simulink model "qpsk_phase_uw"  (R2016b)
settings: Solver=VariableStepAuto  StartTime=0.0  StopTime=(12+8+84)*8*4-1  RelTol=1e-3  EnableMultiTasking=on
undefined symbols (not defined in the file or in its folder): jsin, K1, K2, rcosine
libraries: dspstat3 x1
settings Model: Creator=coltmt  LastModifiedBy=colttom
settings DataIOCC: LimitDataPoints=on
settings OptimizationCC: LifeSpan=inf
settings DebuggingCC: AllowSymbolicDim=off  SFUnexpectedBacktrackingDiag=warning  SFNoUnconditionalDefaultTransitionDiag=warning  SFExecutionAtInitializationDiag=none
settings ModelReferenceCC: PropagateSignalLabelsOutOfModel=off
settings GRTTargetCC: TargetLangStandard=C89/C90 (ANSI)
settings ConfigComp: CovMetricSettings=dw  CovHtmlReporting=on  CovSaveCumulativeToWorkspaceVar=on  CovSaveSingleToWorkspaceVar=on  CovExternalEMLEnable=off

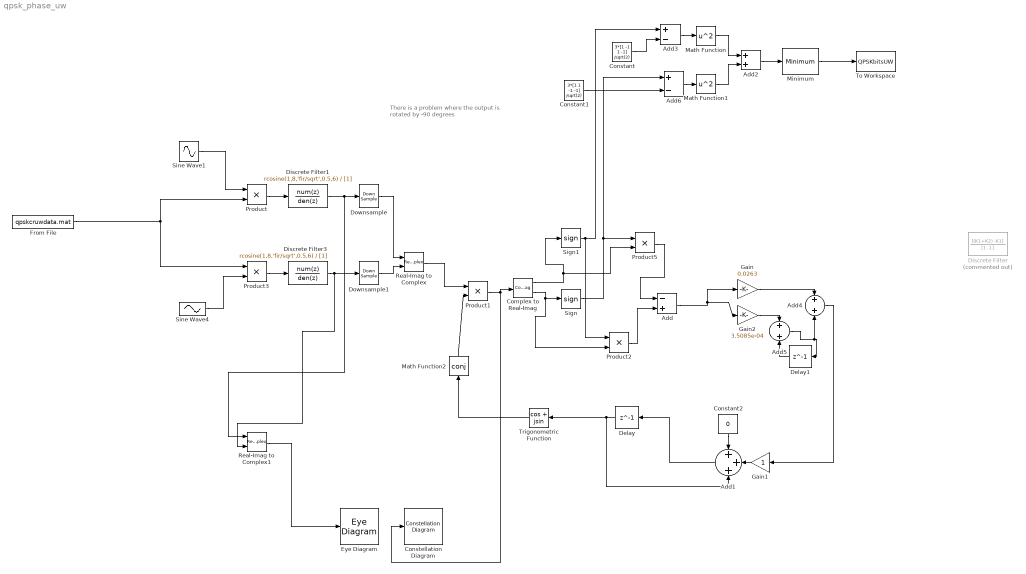
== system qpsk_phase_uw ==
  note: There is a problem where the output is
      | rotated by -90 degrees
  Add : Sum  Inputs=-+
  Add1 : Sum  Inputs=+++
  Add2 : Sum
  Add3 : Sum  Inputs=+-
  Add4 : Sum
  Add5 : Sum
  Add6 : Sum  Inputs=+-
  Complex to Real-Imag : ComplexToRealImag
  Constant : Constant  Value=3*[1 -1 1 -1] /sqrt(2)
  Constant1 : Constant  Value=3*[1 1 -1 -1] /sqrt(2)
  Constant2 : Constant  Value=0
  Constellation Diagram : ConstellationDiagram
  Delay : Delay  DelayLength=1
  Delay1 : Delay  DelayLength=1
  Discrete Filter : DiscreteFilter  Commented=on  Numerator=[(K1+K2) -K1]  Denominator=[1 -1]
  Discrete Filter1 : DiscreteFilter  Numerator=rcosine(1,8,'fir/sqrt',0.5,6)  Denominator=[1]
  Discrete Filter3 : DiscreteFilter  Numerator=rcosine(1,8,'fir/sqrt',0.5,6)  Denominator=[1]
  Downsample : DownSample  N=8  InputProcessing=Inherited (this choice will be removed - see release notes)  RateOptions=Allow multirate processing
  Downsample1 : DownSample  N=8  InputProcessing=Inherited (this choice will be removed - see release notes)  RateOptions=Allow multirate processing
  Eye Diagram : EyeDiagram
  From File : FromFile  FileName=qpskcruwdata.mat
  Gain : Gain  Gain=0.0263
  Gain1 : Gain
  Gain2 : Gain  Gain=3.5085e-04
  Math Function : Math  Operator=square  SaturateOnIntegerOverflow=on
  Math Function1 : Math  Operator=square  SaturateOnIntegerOverflow=on
  Math Function2 : Math  Operator=conj  SaturateOnIntegerOverflow=on
  Minimum : dspstat3/Minimum  operation=minimum  fcn=Index  indexBase=Zero  operateOver=Each column  Dimension=1  InputProcessing=Columns as channels (frame based)  reset=None  roiEnable=off  roiType=Rectangles  roiPortion=Entire ROI  roiOutput=Individual statistics for each ROI  roiFlag=off  roundingMode=Floor  overflowMode=off
  Product{,1..3,5} (5 alike) : Product
  Real-Imag to Complex : RealImagToComplex
  Real-Imag to Complex1 : RealImagToComplex
  Sign : Signum
  Sign1 : Signum
  Sine Wave1 : Sin  Amplitude=sqrt(2)  Frequency=.3*2*pi  Phase=pi/2  SampleTime=1
  Sine Wave4 : Sin  Amplitude=-sqrt(2)  Frequency=.3*2*pi  SampleTime=1
  To Workspace : ToWorkspace  VariableName=QPSKbitsUW  SampleTime=-1
  Trigonometric Function : Trigonometry  Operator=cos + jsin
  wires:
  Constant2/1 -> Add1/1
  Add1/1 -> Delay/1
  Delay/1 -> Trigonometric Function/1, Add1/3
  Gain1/1 -> Add1/2
  Trigonometric Function/1 -> Math Function2/1
  Sine Wave1/1 -> Product/1
  Sine Wave4/1 -> Product3/2
  Product/1 -> Discrete Filter1/1
  Product3/1 -> Discrete Filter3/1
  Discrete Filter1/1 -> Real-Imag to Complex1/1, Downsample/1
  From File/1 -> Product/2, Product3/1
  Complex to Real-Imag/2 -> Product2/2, Sign/1
  Discrete Filter3/1 -> Real-Imag to Complex1/2, Downsample1/1
  Real-Imag to Complex1/1 -> Eye Diagram/1
  Gain/1 -> Add4/1
  Delay1/1 -> Add5/2
  Add5/1 -> Delay1/1, Add4/2
  Gain2/1 -> Add5/1
  Math Function2/1 -> Product1/2
  Product5/1 -> Add/1
  Product2/1 -> Add/2
  Downsample/1 -> Real-Imag to Complex/1
  Downsample1/1 -> Real-Imag to Complex/2
  Real-Imag to Complex/1 -> Product1/1
  Complex to Real-Imag/1 -> Sign1/1, Product5/2
  Sign1/1 -> Add3/1, Product2/1
  Sign/1 -> Add6/1, Product5/1
  Math Function/1 -> Add2/1
  Math Function1/1 -> Add2/2
  Product1/1 -> Complex to Real-Imag/1, Constellation Diagram/1
  Add3/1 -> Math Function/1
  Add6/1 -> Math Function1/1
  Constant/1 -> Add3/2
  Constant1/1 -> Add6/2
  Add2/1 -> Minimum/1
  Minimum/1 -> To Workspace/1
  Add/1 -> Gain2/1, Gain/1
  Add4/1 -> Gain1/1
